simulink model "Dan_model2b"  (Simulink 7.8)
settings: Solver=ode45  StartTime=0.0  StopTime=10.0  RelTol=1e-3
values from neighbouring files (symbols this model uses):
  a = avect(i)    [ps7-p1.m]    (also in ps7-task2.m = -1)
  K = minreal(K_vec)    [ps7-task3.m]
settings Model: Creator=Dan  LastModifiedBy=Dan
settings DebuggingCC: InitInArrayFormatMsg=none

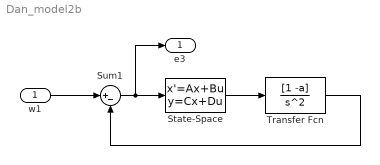
== system Dan_model2b ==
  w1 : Inport
  State-Space : StateSpace  A=K.A  B=K.B  C=K.C  D=K.D
  Sum1 : Sum  Inputs=|+-
  Transfer Fcn : TransferFcn  Numerator=[1 -a]  Denominator=[1 0 0]
  e3 : Outport
  wires:
  w1/1 -> Sum1/1
  Transfer Fcn/1 -> Sum1/2
  Sum1/1 -> State-Space/1, e3/1
  State-Space/1 -> Transfer Fcn/1
